simulink model "tarefa1_modelo2"  (R2012b)
settings: Solver=ode45  StartTime=0.0  StopTime=10.0  RelTol=1e-3
values from neighbouring files (symbols this model uses):
  K = 0.02    [Controle_Lab4.m]    (also in Lab8.m = place(A,B,[-10 -12 -2]); Tarefa1.m)
  Kp = Kkp/K    (= 358.333333333)    [Controle_Lab4.m]    (also in Tarefa1.m = 300)
  L = 1.024 - Start    (= 0.024)    [Controle_Lab4.m]    (also in Tarefa1.m = 0.03)
  T = 1.196 - L - Start    (= 0.172)    [Controle_Lab4.m]    (also in Tarefa1.m = 0.18)
settings Model: Creator=11104980  LastModifiedBy=11104980

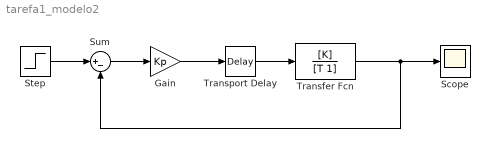
== system tarefa1_modelo2 ==
  Gain : Gain  Gain=Kp
  Scope : Scope
      settings: SaveName=y
  Step : Step  SampleTime=0
  Sum : Sum  Inputs=|+-
  Transfer Fcn : TransferFcn  Numerator=[K]  Denominator=[T 1]
  Transport Delay : TransportDelay  DelayTime=L
  wires:
  Transport Delay/1 -> Transfer Fcn/1
  Gain/1 -> Transport Delay/1
  Sum/1 -> Gain/1
  Transfer Fcn/1 -> Scope/1, Sum/2
  Step/1 -> Sum/1
